simulink model "untitled"  (R2018a)
settings: Solver=FixedStepDiscrete  StartTime=0.0  StopTime=100  RelTol=1e-3
values from neighbouring files (symbols this model uses):
  coeff = randi([0, 1], 3, 60)*2-1    [Untitled.m]
libraries: filter_library x261, simulink x2, dspsrcs4 x1
(part 1 of 2)
settings Model: Creator=Orion  LastModifiedBy=Orion
settings OptimizationCC: BlockReduction=off  ConditionallyExecuteInputs=off  DefaultParameterBehavior=Inlined
settings DebuggingCC: AlgebraicLoopMsg=error  SingleTaskRateTransMsg=error
settings HardwareCC: ProdBitPerPointer=32  ProdBitPerSizeT=32  ProdBitPerPtrDiffT=32  ProdLargestAtomicFloat=None  ProdIntDivRoundTo=Undefined  ProdEndianess=Unspecified  ProdWordSize=32  ProdHWDeviceType=ASIC/FPGA->ASIC/FPGA  TargetBitPerPointer=64  TargetBitPerSizeT=64  TargetBitPerPtrDiffT=64  TargetLongLongMode=on  TargetIntDivRoundTo=Zero  TargetEndianess=LittleEndian  TargetWordSize=64  TargetHWDeviceType=Custom Processor->MATLAB Host Computer  ProdEqTarget=off

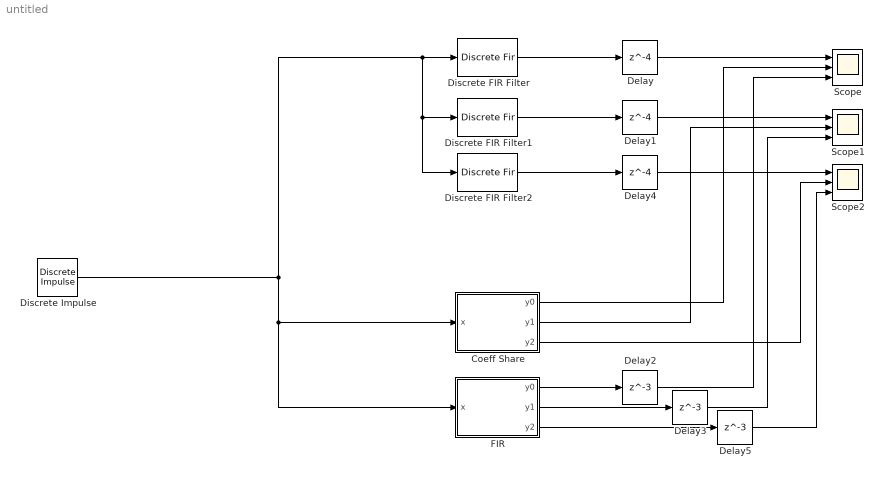
== system untitled ==
  Coeff Share : Subsystem
  Delay : Delay  DelayLength=4  InitialCondition=0
  Delay1 : Delay  DelayLength=4  InitialCondition=0
  Delay2 : Delay  DelayLength=3  InitialCondition=0
  Delay3 : Delay  DelayLength=3  InitialCondition=0
  Delay4 : Delay  DelayLength=4  InitialCondition=0
  Delay5 : Delay  DelayLength=3  InitialCondition=0
  Discrete Impulse : dspsrcs4/Discrete  Impulse  Delay=0  SampleTime=1  FrameSample=1  OutputFrames=off  dataType=Fixed-point  isSigned=on  wordLen=12  udDataType=sfix(16)  fracBitsMode=User-defined  numFracBits=11  OutDataTypeStr=fixdt(1,12,11)  LastOutDataTypeStr=fixdt(1,12,11)
  Discrete FIR Filter : DiscreteFir  Coefficients=coeff(1, :)
  Discrete FIR Filter1 : DiscreteFir  Coefficients=coeff(2, :)
  Discrete FIR Filter2 : DiscreteFir  Coefficients=coeff(3, :)
  FIR : Subsystem
  Scope : Scope  NumInputPorts=3
  Scope1 : Scope  NumInputPorts=3
  Scope2 : Scope  NumInputPorts=3
  wires:
  Discrete Impulse/1 -> FIR/1(x), Coeff Share/1(x), Discrete FIR Filter2/1, Discrete FIR Filter1/1, Discrete FIR Filter/1
  Discrete FIR Filter/1 -> Delay/1
  Delay/1 -> Scope/1
  Discrete FIR Filter1/1 -> Delay1/1
  Delay1/1 -> Scope1/1
  Coeff Share/1(y0) -> Scope/2
  Coeff Share/2(y1) -> Scope1/2
  FIR/1(y0) -> Delay2/1
  FIR/2(y1) -> Delay3/1
  Delay2/1 -> Scope/3
  Delay3/1 -> Scope1/3
  Discrete FIR Filter2/1 -> Delay4/1
  Delay4/1 -> Scope2/1
  Coeff Share/3(y2) -> Scope2/2
  FIR/3(y2) -> Delay5/1
  Delay5/1 -> Scope2/3

== system untitled/Coeff Share ==
  x : Inport
  Filter 0 : Subsystem
  Filter 1 : Subsystem
  Filter 2 : Subsystem
  Multiply-Accumulate 0 : Subsystem
  Multiply-Accumulate 1 : Subsystem
  Multiply-Accumulate 2 : Subsystem
  Multiply-Accumulate 3 : Subsystem
  Multiply-Accumulate 4 : Subsystem
  Multiply-Accumulate 5 : Subsystem
  Multiply-Accumulate 6 : Subsystem
  Multiply-Accumulate 7 : Subsystem
  Mux : Mux  Inputs=8
  Tapped Delay Line : simulink/Discrete/Tapped Delay  vinit=0.0  samptime=-1  NumDelays=60  DelayOrder=Newest  includeCurrent=off
  y0 : Outport
  y1 : Outport  Port=2
  y2 : Outport  Port=3
  wires:
  x/1 -> Tapped Delay Line/1
  Tapped Delay Line/1 -> Multiply-Accumulate 0/1(x), Multiply-Accumulate 1/1(x), Multiply-Accumulate 2/1(x), Multiply-Accumulate 3/1(x), Multiply-Accumulate 4/1(x), Multiply-Accumulate 5/1(x), Multiply-Accumulate 6/1(x), Multiply-Accumulate 7/1(x)
  Multiply-Accumulate 0/1(y) -> Mux/1
  Multiply-Accumulate 1/1(y) -> Mux/2
  Multiply-Accumulate 2/1(y) -> Mux/3
  Multiply-Accumulate 3/1(y) -> Mux/4
  Multiply-Accumulate 4/1(y) -> Mux/5
  Multiply-Accumulate 5/1(y) -> Mux/6
  Multiply-Accumulate 6/1(y) -> Mux/7
  Multiply-Accumulate 7/1(y) -> Mux/8
  Mux/1 -> Filter 0/1(data_in), Filter 1/1(data_in), Filter 2/1(data_in)
  Filter 0/1(data_out) -> y0/1
  Filter 1/1(data_out) -> y1/1
  Filter 2/1(data_out) -> y2/1

== system untitled/FIR ==
  x : Inport
  Multiply-Accumulate 1 : Subsystem
  Multiply-Accumulate 2 : Subsystem
  Multiply-Accumulate 3 : Subsystem
  Tapped Delay Line : simulink/Discrete/Tapped Delay  vinit=0.0  samptime=-1  NumDelays=60  DelayOrder=Newest  includeCurrent=off
  y0 : Outport
  y1 : Outport  Port=2
  y2 : Outport  Port=3
  wires:
  x/1 -> Tapped Delay Line/1
  Tapped Delay Line/1 -> Multiply-Accumulate 1/1(x), Multiply-Accumulate 2/1(x), Multiply-Accumulate 3/1(x)
  Multiply-Accumulate 1/1(y) -> y0/1
  Multiply-Accumulate 2/1(y) -> y1/1
  Multiply-Accumulate 3/1(y) -> y2/1

== system untitled/Coeff Share/Filter 0 ==
  data_in : Inport
  Demux : Demux  Outputs=8
  add_delay1_{1..4} (4 alike) : filter_library/Add and Delay  Inputs=++
      settings: SourceProductName=Filter Library
  add_delay2_1 : filter_library/Add and Delay  Inputs=++
      settings: SourceProductName=Filter Library
  add_delay2_2 : filter_library/Add and Delay  Inputs=++
      settings: SourceProductName=Filter Library
  add_delay3_1 : filter_library/Add and Delay  Inputs=++
      settings: SourceProductName=Filter Library
  data_out : Outport
  wires:
  add_delay1_1/1 -> add_delay2_1/1
  add_delay1_2/1 -> add_delay2_1/2
  add_delay1_3/1 -> add_delay2_2/1
  add_delay1_4/1 -> add_delay2_2/2
  add_delay2_1/1 -> add_delay3_1/1
  add_delay2_2/1 -> add_delay3_1/2
  Demux/1 -> add_delay1_1/1
  Demux/2 -> add_delay1_1/2
  Demux/3 -> add_delay1_2/1
  Demux/4 -> add_delay1_2/2
  Demux/5 -> add_delay1_3/1
  Demux/6 -> add_delay1_3/2
  Demux/7 -> add_delay1_4/1
  Demux/8 -> add_delay1_4/2
  add_delay3_1/1 -> data_out/1
  data_in/1 -> Demux/1

== system untitled/Coeff Share/Filter 1 ==
  data_in : Inport
  Demux : Demux  Outputs=8
  add_delay1_1 : filter_library/Add and Delay  Inputs=++
      settings: SourceProductName=Filter Library
  add_delay1_2 : filter_library/Add and Delay  Inputs=--
      settings: SourceProductName=Filter Library
  add_delay1_3 : filter_library/Add and Delay  Inputs=--
      settings: SourceProductName=Filter Library
  add_delay1_4 : filter_library/Add and Delay  Inputs=++
      settings: SourceProductName=Filter Library
  add_delay2_1 : filter_library/Add and Delay  Inputs=++
      settings: SourceProductName=Filter Library
  add_delay2_2 : filter_library/Add and Delay  Inputs=++
      settings: SourceProductName=Filter Library
  add_delay3_1 : filter_library/Add and Delay  Inputs=++
      settings: SourceProductName=Filter Library
  data_out : Outport
  wires:
  add_delay1_1/1 -> add_delay2_1/1
  add_delay1_2/1 -> add_delay2_1/2
  add_delay1_3/1 -> add_delay2_2/1
  add_delay1_4/1 -> add_delay2_2/2
  add_delay2_1/1 -> add_delay3_1/1
  add_delay2_2/1 -> add_delay3_1/2
  Demux/1 -> add_delay1_1/1
  Demux/2 -> add_delay1_1/2
  Demux/3 -> add_delay1_2/1
  Demux/4 -> add_delay1_2/2
  Demux/5 -> add_delay1_3/1
  Demux/6 -> add_delay1_3/2
  Demux/7 -> add_delay1_4/1
  Demux/8 -> add_delay1_4/2
  add_delay3_1/1 -> data_out/1
  data_in/1 -> Demux/1

== system untitled/Coeff Share/Filter 2 ==
  data_in : Inport
  Demux : Demux  Outputs=8
  add_delay1_1 : filter_library/Add and Delay  Inputs=+-
      settings: SourceProductName=Filter Library
  add_delay1_2 : filter_library/Add and Delay  Inputs=+-
      settings: SourceProductName=Filter Library
  add_delay1_3 : filter_library/Add and Delay  Inputs=-+
      settings: SourceProductName=Filter Library
  add_delay1_4 : filter_library/Add and Delay  Inputs=-+
      settings: SourceProductName=Filter Library
  add_delay2_1 : filter_library/Add and Delay  Inputs=++
      settings: SourceProductName=Filter Library
  add_delay2_2 : filter_library/Add and Delay  Inputs=++
      settings: SourceProductName=Filter Library
  add_delay3_1 : filter_library/Add and Delay  Inputs=++
      settings: SourceProductName=Filter Library
  data_out : Outport
  wires:
  add_delay1_1/1 -> add_delay2_1/1
  add_delay1_2/1 -> add_delay2_1/2
  add_delay1_3/1 -> add_delay2_2/1
  add_delay1_4/1 -> add_delay2_2/2
  add_delay2_1/1 -> add_delay3_1/1
  add_delay2_2/1 -> add_delay3_1/2
  Demux/1 -> add_delay1_1/1
  Demux/2 -> add_delay1_1/2
  Demux/3 -> add_delay1_2/1
  Demux/4 -> add_delay1_2/2
  Demux/5 -> add_delay1_3/1
  Demux/6 -> add_delay1_3/2
  Demux/7 -> add_delay1_4/1
  Demux/8 -> add_delay1_4/2
  add_delay3_1/1 -> data_out/1
  data_in/1 -> Demux/1

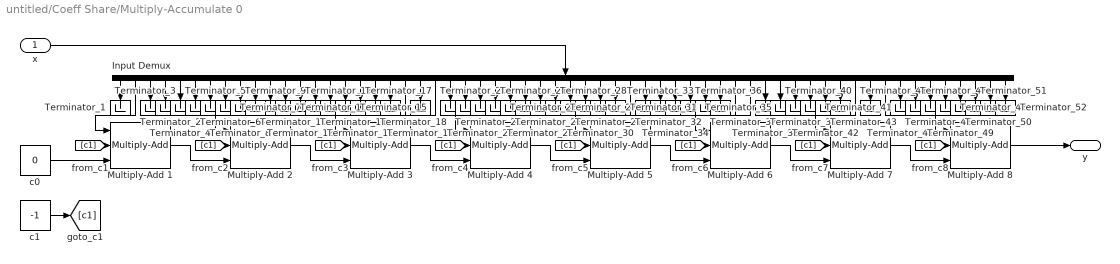
== system untitled/Coeff Share/Multiply-Accumulate 0 ==
  x : Inport
  Input Demux : Demux  Outputs=60
  Multiply-Add {1..8} (8 alike) : filter_library/Multiply-Add  SystemSampleTime=-1
      settings: SourceProductName=Filter Library
  Terminator_{1..52} (52 alike) : Terminator
  c0 : Constant  Value=0  OutDataTypeStr=fixdt(1, 12, 7)  SampleTime=1
  c1 : Constant  Value=-1  OutDataTypeStr=fixdt(1, 12, 7)  SampleTime=1
  y : Outport
  wires:
  [c1] -> Multiply-Add 1/2
  [c1] -> Multiply-Add 2/2
  [c1] -> Multiply-Add 3/2
  [c1] -> Multiply-Add 4/2
  [c1] -> Multiply-Add 5/2
  [c1] -> Multiply-Add 6/2
  [c1] -> Multiply-Add 7/2
  [c1] -> Multiply-Add 8/2
  Multiply-Add 1/1 -> Multiply-Add 2/3
  Multiply-Add 2/1 -> Multiply-Add 3/3
  Multiply-Add 3/1 -> Multiply-Add 4/3
  Multiply-Add 4/1 -> Multiply-Add 5/3
  Multiply-Add 5/1 -> Multiply-Add 6/3
  Multiply-Add 6/1 -> Multiply-Add 7/3
  Multiply-Add 7/1 -> Multiply-Add 8/3
  Multiply-Add 8/1 -> y/1
  x/1 -> Input Demux/1
  Input Demux/2 -> Multiply-Add 1/1
  Input Demux/20 -> Multiply-Add 2/1
  Input Demux/22 -> Multiply-Add 3/1
  Input Demux/35 -> Multiply-Add 4/1
  Input Demux/42 -> Multiply-Add 5/1
  Input Demux/43 -> Multiply-Add 6/1
  Input Demux/50 -> Multiply-Add 7/1
  Input Demux/52 -> Multiply-Add 8/1
  c1/1 -> [c1]
  c0/1 -> Multiply-Add 1/3
  Input Demux/1 -> Terminator_1/1
  Input Demux/3 -> Terminator_2/1
  Input Demux/4 -> Terminator_3/1
  Input Demux/5 -> Terminator_4/1
  Input Demux/6 -> Terminator_5/1
  Input Demux/7 -> Terminator_6/1
  Input Demux/8 -> Terminator_7/1
  Input Demux/9 -> Terminator_8/1
  Input Demux/10 -> Terminator_9/1
  Input Demux/11 -> Terminator_10/1
  Input Demux/12 -> Terminator_11/1
  Input Demux/13 -> Terminator_12/1
  Input Demux/14 -> Terminator_13/1
  Input Demux/15 -> Terminator_14/1
  Input Demux/16 -> Terminator_15/1
  Input Demux/17 -> Terminator_16/1
  Input Demux/18 -> Terminator_17/1
  Input Demux/19 -> Terminator_18/1
  Input Demux/21 -> Terminator_19/1
  Input Demux/23 -> Terminator_20/1
  Input Demux/24 -> Terminator_21/1
  Input Demux/25 -> Terminator_22/1
  Input Demux/26 -> Terminator_23/1
  Input Demux/27 -> Terminator_24/1
  Input Demux/28 -> Terminator_25/1
  Input Demux/29 -> Terminator_26/1
  Input Demux/30 -> Terminator_27/1
  Input Demux/31 -> Terminator_28/1
  Input Demux/32 -> Terminator_29/1
  Input Demux/33 -> Terminator_30/1
  Input Demux/34 -> Terminator_31/1
  Input Demux/36 -> Terminator_32/1
  Input Demux/37 -> Terminator_33/1
  Input Demux/38 -> Terminator_34/1
  Input Demux/39 -> Terminator_35/1
  Input Demux/40 -> Terminator_36/1
  Input Demux/41 -> Terminator_37/1
  Input Demux/44 -> Terminator_38/1
  Input Demux/45 -> Terminator_39/1
  Input Demux/46 -> Terminator_40/1
  Input Demux/47 -> Terminator_41/1
  Input Demux/48 -> Terminator_42/1
  Input Demux/49 -> Terminator_43/1
  Input Demux/51 -> Terminator_44/1
  Input Demux/53 -> Terminator_45/1
  Input Demux/54 -> Terminator_46/1
  Input Demux/55 -> Terminator_47/1
  Input Demux/56 -> Terminator_48/1
  Input Demux/57 -> Terminator_49/1
  Input Demux/58 -> Terminator_50/1
  Input Demux/59 -> Terminator_51/1
  Input Demux/60 -> Terminator_52/1

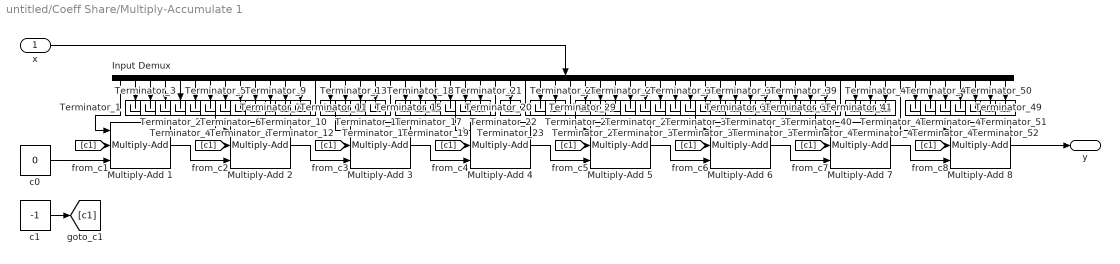
== system untitled/Coeff Share/Multiply-Accumulate 1 ==
  x : Inport
  Input Demux : Demux  Outputs=60
  Multiply-Add {1..8} (8 alike) : filter_library/Multiply-Add  SystemSampleTime=-1
      settings: SourceProductName=Filter Library
  Terminator_{1..52} (52 alike) : Terminator
  c0 : Constant  Value=0  OutDataTypeStr=fixdt(1, 12, 7)  SampleTime=1
  c1 : Constant  Value=-1  OutDataTypeStr=fixdt(1, 12, 7)  SampleTime=1
  y : Outport
  wires:
  [c1] -> Multiply-Add 1/2
  [c1] -> Multiply-Add 2/2
  [c1] -> Multiply-Add 3/2
  [c1] -> Multiply-Add 4/2
  [c1] -> Multiply-Add 5/2
  [c1] -> Multiply-Add 6/2
  [c1] -> Multiply-Add 7/2
  [c1] -> Multiply-Add 8/2
  Multiply-Add 1/1 -> Multiply-Add 2/3
  Multiply-Add 2/1 -> Multiply-Add 3/3
  Multiply-Add 3/1 -> Multiply-Add 4/3
  Multiply-Add 4/1 -> Multiply-Add 5/3
  Multiply-Add 5/1 -> Multiply-Add 6/3
  Multiply-Add 6/1 -> Multiply-Add 7/3
  Multiply-Add 7/1 -> Multiply-Add 8/3
  Multiply-Add 8/1 -> y/1
  x/1 -> Input Demux/1
  Input Demux/1 -> Multiply-Add 1/1
  Input Demux/14 -> Multiply-Add 2/1
  Input Demux/19 -> Multiply-Add 3/1
  Input Demux/26 -> Multiply-Add 4/1
  Input Demux/28 -> Multiply-Add 5/1
  Input Demux/31 -> Multiply-Add 6/1
  Input Demux/49 -> Multiply-Add 7/1
  Input Demux/53 -> Multiply-Add 8/1
  c1/1 -> [c1]
  c0/1 -> Multiply-Add 1/3
  Input Demux/2 -> Terminator_1/1
  Input Demux/3 -> Terminator_2/1
  Input Demux/4 -> Terminator_3/1
  Input Demux/5 -> Terminator_4/1
  Input Demux/6 -> Terminator_5/1
  Input Demux/7 -> Terminator_6/1
  Input Demux/8 -> Terminator_7/1
  Input Demux/9 -> Terminator_8/1
  Input Demux/10 -> Terminator_9/1
  Input Demux/11 -> Terminator_10/1
  Input Demux/12 -> Terminator_11/1
  Input Demux/13 -> Terminator_12/1
  Input Demux/15 -> Terminator_13/1
  Input Demux/16 -> Terminator_14/1
  Input Demux/17 -> Terminator_15/1
  Input Demux/18 -> Terminator_16/1
  Input Demux/20 -> Terminator_17/1
  Input Demux/21 -> Terminator_18/1
  Input Demux/22 -> Terminator_19/1
  Input Demux/23 -> Terminator_20/1
  Input Demux/24 -> Terminator_21/1
  Input Demux/25 -> Terminator_22/1
  Input Demux/27 -> Terminator_23/1
  Input Demux/29 -> Terminator_24/1
  Input Demux/30 -> Terminator_25/1
  Input Demux/32 -> Terminator_26/1
  Input Demux/33 -> Terminator_27/1
  Input Demux/34 -> Terminator_28/1
  Input Demux/35 -> Terminator_29/1
  Input Demux/36 -> Terminator_30/1
  Input Demux/37 -> Terminator_31/1
  Input Demux/38 -> Terminator_32/1
  Input Demux/39 -> Terminator_33/1
  Input Demux/40 -> Terminator_34/1
  Input Demux/41 -> Terminator_35/1
  Input Demux/42 -> Terminator_36/1
  Input Demux/43 -> Terminator_37/1
  Input Demux/44 -> Terminator_38/1
  Input Demux/45 -> Terminator_39/1
  Input Demux/46 -> Terminator_40/1
  Input Demux/47 -> Terminator_41/1
  Input Demux/48 -> Terminator_42/1
  Input Demux/50 -> Terminator_43/1
  Input Demux/51 -> Terminator_44/1
  Input Demux/52 -> Terminator_45/1
  Input Demux/54 -> Terminator_46/1
  Input Demux/55 -> Terminator_47/1
  Input Demux/56 -> Terminator_48/1
  Input Demux/57 -> Terminator_49/1
  Input Demux/58 -> Terminator_50/1
  Input Demux/59 -> Terminator_51/1
  Input Demux/60 -> Terminator_52/1

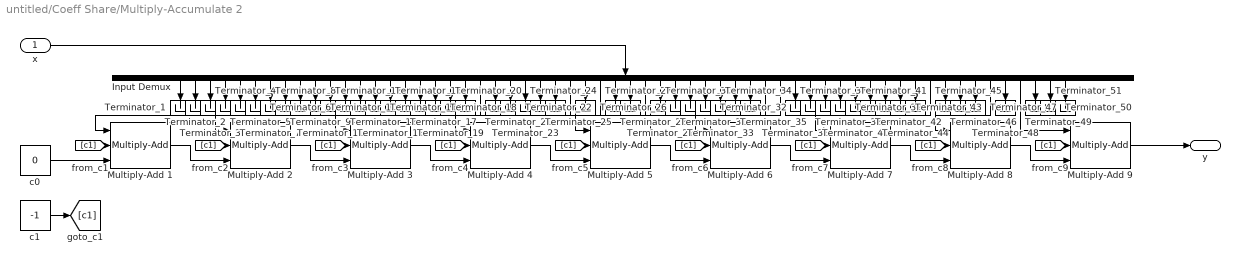
== system untitled/Coeff Share/Multiply-Accumulate 2 ==
  x : Inport
  Input Demux : Demux  Outputs=60
  Multiply-Add {1..9} (9 alike) : filter_library/Multiply-Add  SystemSampleTime=-1
      settings: SourceProductName=Filter Library
  Terminator_{1..51} (51 alike) : Terminator
  c0 : Constant  Value=0  OutDataTypeStr=fixdt(1, 12, 7)  SampleTime=1
  c1 : Constant  Value=-1  OutDataTypeStr=fixdt(1, 12, 7)  SampleTime=1
  y : Outport
  wires:
  [c1] -> Multiply-Add 1/2
  [c1] -> Multiply-Add 2/2
  [c1] -> Multiply-Add 3/2
  [c1] -> Multiply-Add 4/2
  [c1] -> Multiply-Add 5/2
  [c1] -> Multiply-Add 6/2
  [c1] -> Multiply-Add 7/2
  [c1] -> Multiply-Add 8/2
  [c1] -> Multiply-Add 9/2
  Multiply-Add 1/1 -> Multiply-Add 2/3
  Multiply-Add 2/1 -> Multiply-Add 3/3
  Multiply-Add 3/1 -> Multiply-Add 4/3
  Multiply-Add 4/1 -> Multiply-Add 5/3
  Multiply-Add 5/1 -> Multiply-Add 6/3
  Multiply-Add 6/1 -> Multiply-Add 7/3
  Multiply-Add 7/1 -> Multiply-Add 8/3
  Multiply-Add 8/1 -> Multiply-Add 9/3
  Multiply-Add 9/1 -> y/1
  x/1 -> Input Demux/1
  Input Demux/21 -> Multiply-Add 1/1
  Input Demux/27 -> Multiply-Add 2/1
  Input Demux/29 -> Multiply-Add 3/1
  Input Demux/32 -> Multiply-Add 4/1
  Input Demux/40 -> Multiply-Add 5/1
  Input Demux/41 -> Multiply-Add 6/1
  Input Demux/51 -> Multiply-Add 7/1
  Input Demux/55 -> Multiply-Add 8/1
  Input Demux/57 -> Multiply-Add 9/1
  c1/1 -> [c1]
  c0/1 -> Multiply-Add 1/3
  Input Demux/1 -> Terminator_1/1
  Input Demux/2 -> Terminator_2/1
  Input Demux/3 -> Terminator_3/1
  Input Demux/4 -> Terminator_4/1
  Input Demux/5 -> Terminator_5/1
  Input Demux/6 -> Terminator_6/1
  Input Demux/7 -> Terminator_7/1
  Input Demux/8 -> Terminator_8/1
  Input Demux/9 -> Terminator_9/1
  Input Demux/10 -> Terminator_10/1
  Input Demux/11 -> Terminator_11/1
  Input Demux/12 -> Terminator_12/1
  Input Demux/13 -> Terminator_13/1
  Input Demux/14 -> Terminator_14/1
  Input Demux/15 -> Terminator_15/1
  Input Demux/16 -> Terminator_16/1
  Input Demux/17 -> Terminator_17/1
  Input Demux/18 -> Terminator_18/1
  Input Demux/19 -> Terminator_19/1
  Input Demux/20 -> Terminator_20/1
  Input Demux/22 -> Terminator_21/1
  Input Demux/23 -> Terminator_22/1
  Input Demux/24 -> Terminator_23/1
  Input Demux/25 -> Terminator_24/1
  Input Demux/26 -> Terminator_25/1
  Input Demux/28 -> Terminator_26/1
  Input Demux/30 -> Terminator_27/1
  Input Demux/31 -> Terminator_28/1
  Input Demux/33 -> Terminator_29/1
  Input Demux/34 -> Terminator_30/1
  Input Demux/35 -> Terminator_31/1
  Input Demux/36 -> Terminator_32/1
  Input Demux/37 -> Terminator_33/1
  Input Demux/38 -> Terminator_34/1
  Input Demux/39 -> Terminator_35/1
  Input Demux/42 -> Terminator_36/1
  Input Demux/43 -> Terminator_37/1
  Input Demux/44 -> Terminator_38/1
  Input Demux/45 -> Terminator_39/1
  Input Demux/46 -> Terminator_40/1
  Input Demux/47 -> Terminator_41/1
  Input Demux/48 -> Terminator_42/1
  Input Demux/49 -> Terminator_43/1
  Input Demux/50 -> Terminator_44/1
  Input Demux/52 -> Terminator_45/1
  Input Demux/53 -> Terminator_46/1
  Input Demux/54 -> Terminator_47/1
  Input Demux/56 -> Terminator_48/1
  Input Demux/58 -> Terminator_49/1
  Input Demux/59 -> Terminator_50/1
  Input Demux/60 -> Terminator_51/1

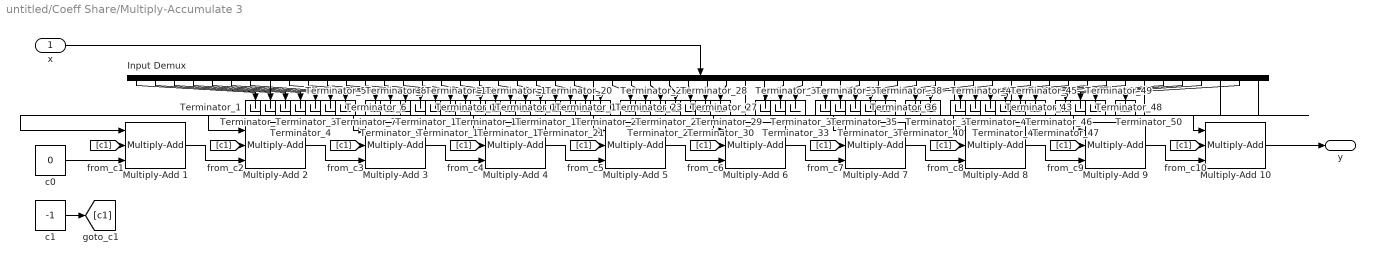
== system untitled/Coeff Share/Multiply-Accumulate 3 ==
  x : Inport
  Input Demux : Demux  Outputs=60
  Multiply-Add {1..10} (10 alike) : filter_library/Multiply-Add  SystemSampleTime=-1
      settings: SourceProductName=Filter Library
  Terminator_{1..50} (50 alike) : Terminator
  c0 : Constant  Value=0  OutDataTypeStr=fixdt(1, 12, 7)  SampleTime=1
  c1 : Constant  Value=-1  OutDataTypeStr=fixdt(1, 12, 7)  SampleTime=1
  y : Outport
  wires:
  [c1] -> Multiply-Add 1/2
  [c1] -> Multiply-Add 2/2
  [c1] -> Multiply-Add 3/2
  [c1] -> Multiply-Add 4/2
  [c1] -> Multiply-Add 5/2
  [c1] -> Multiply-Add 6/2
  [c1] -> Multiply-Add 7/2
  [c1] -> Multiply-Add 8/2
  [c1] -> Multiply-Add 9/2
  [c1] -> Multiply-Add 10/2
  Multiply-Add 1/1 -> Multiply-Add 2/3
  Multiply-Add 2/1 -> Multiply-Add 3/3
  Multiply-Add 3/1 -> Multiply-Add 4/3
  Multiply-Add 4/1 -> Multiply-Add 5/3
  Multiply-Add 5/1 -> Multiply-Add 6/3
  Multiply-Add 6/1 -> Multiply-Add 7/3
  Multiply-Add 7/1 -> Multiply-Add 8/3
  Multiply-Add 8/1 -> Multiply-Add 9/3
  Multiply-Add 9/1 -> Multiply-Add 10/3
  Multiply-Add 10/1 -> y/1
  x/1 -> Input Demux/1
  Input Demux/8 -> Multiply-Add 1/1
  Input Demux/25 -> Multiply-Add 2/1
  Input Demux/33 -> Multiply-Add 3/1
  Input Demux/34 -> Multiply-Add 4/1
  Input Demux/38 -> Multiply-Add 5/1
  Input Demux/44 -> Multiply-Add 6/1
  Input Demux/47 -> Multiply-Add 7/1
  Input Demux/54 -> Multiply-Add 8/1
  Input Demux/58 -> Multiply-Add 9/1
  Input Demux/60 -> Multiply-Add 10/1
  c1/1 -> [c1]
  c0/1 -> Multiply-Add 1/3
  Input Demux/1 -> Terminator_1/1
  Input Demux/2 -> Terminator_2/1
  Input Demux/3 -> Terminator_3/1
  Input Demux/4 -> Terminator_4/1
  Input Demux/5 -> Terminator_5/1
  Input Demux/6 -> Terminator_6/1
  Input Demux/7 -> Terminator_7/1
  Input Demux/9 -> Terminator_8/1
  Input Demux/10 -> Terminator_9/1
  Input Demux/11 -> Terminator_10/1
  Input Demux/12 -> Terminator_11/1
  Input Demux/13 -> Terminator_12/1
  Input Demux/14 -> Terminator_13/1
  Input Demux/15 -> Terminator_14/1
  Input Demux/16 -> Terminator_15/1
  Input Demux/17 -> Terminator_16/1
  Input Demux/18 -> Terminator_17/1
  Input Demux/19 -> Terminator_18/1
  Input Demux/20 -> Terminator_19/1
  Input Demux/21 -> Terminator_20/1
  Input Demux/22 -> Terminator_21/1
  Input Demux/23 -> Terminator_22/1
  Input Demux/24 -> Terminator_23/1
  Input Demux/26 -> Terminator_24/1
  Input Demux/27 -> Terminator_25/1
  Input Demux/28 -> Terminator_26/1
  Input Demux/29 -> Terminator_27/1
  Input Demux/30 -> Terminator_28/1
  Input Demux/31 -> Terminator_29/1
  Input Demux/32 -> Terminator_30/1
  Input Demux/35 -> Terminator_31/1
  Input Demux/36 -> Terminator_32/1
  Input Demux/37 -> Terminator_33/1
  Input Demux/39 -> Terminator_34/1
  Input Demux/40 -> Terminator_35/1
  Input Demux/41 -> Terminator_36/1
  Input Demux/42 -> Terminator_37/1
  Input Demux/43 -> Terminator_38/1
  Input Demux/45 -> Terminator_39/1
  Input Demux/46 -> Terminator_40/1
  Input Demux/48 -> Terminator_41/1
  Input Demux/49 -> Terminator_42/1
  Input Demux/50 -> Terminator_43/1
  Input Demux/51 -> Terminator_44/1
  Input Demux/52 -> Terminator_45/1
  Input Demux/53 -> Terminator_46/1
  Input Demux/55 -> Terminator_47/1
  Input Demux/56 -> Terminator_48/1
  Input Demux/57 -> Terminator_49/1
  Input Demux/59 -> Terminator_50/1

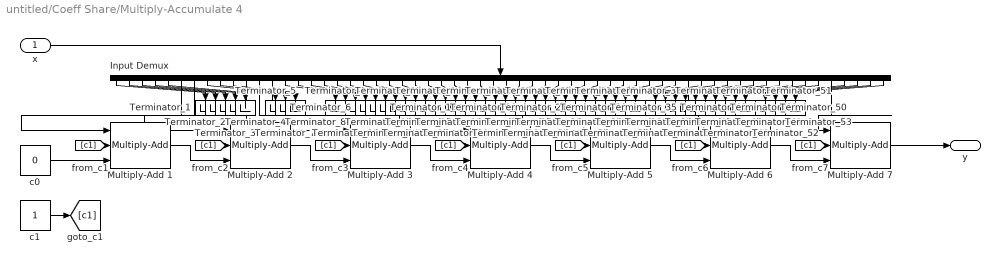
== system untitled/Coeff Share/Multiply-Accumulate 4 ==
  x : Inport
  Input Demux : Demux  Outputs=60
  Multiply-Add {1..7} (7 alike) : filter_library/Multiply-Add  SystemSampleTime=-1
      settings: SourceProductName=Filter Library
  Terminator_{1..53} (53 alike) : Terminator
  c0 : Constant  Value=0  OutDataTypeStr=fixdt(1, 12, 7)  SampleTime=1
  c1 : Constant  OutDataTypeStr=fixdt(1, 12, 7)  SampleTime=1
  y : Outport
  wires:
  [c1] -> Multiply-Add 1/2
  [c1] -> Multiply-Add 2/2
  [c1] -> Multiply-Add 3/2
  [c1] -> Multiply-Add 4/2
  [c1] -> Multiply-Add 5/2
  [c1] -> Multiply-Add 6/2
  [c1] -> Multiply-Add 7/2
  Multiply-Add 1/1 -> Multiply-Add 2/3
  Multiply-Add 2/1 -> Multiply-Add 3/3
  Multiply-Add 3/1 -> Multiply-Add 4/3
  Multiply-Add 4/1 -> Multiply-Add 5/3
  Multiply-Add 5/1 -> Multiply-Add 6/3
  Multiply-Add 6/1 -> Multiply-Add 7/3
  Multiply-Add 7/1 -> y/1
  x/1 -> Input Demux/1
  Input Demux/6 -> Multiply-Add 1/1
  Input Demux/7 -> Multiply-Add 2/1
  Input Demux/11 -> Multiply-Add 3/1
  Input Demux/12 -> Multiply-Add 4/1
  Input Demux/13 -> Multiply-Add 5/1
  Input Demux/45 -> Multiply-Add 6/1
  Input Demux/56 -> Multiply-Add 7/1
  c1/1 -> [c1]
  c0/1 -> Multiply-Add 1/3
  Input Demux/1 -> Terminator_1/1
  Input Demux/2 -> Terminator_2/1
  Input Demux/3 -> Terminator_3/1
  Input Demux/4 -> Terminator_4/1
  Input Demux/5 -> Terminator_5/1
  Input Demux/8 -> Terminator_6/1
  Input Demux/9 -> Terminator_7/1
  Input Demux/10 -> Terminator_8/1
  Input Demux/14 -> Terminator_9/1
  Input Demux/15 -> Terminator_10/1
  Input Demux/16 -> Terminator_11/1
  Input Demux/17 -> Terminator_12/1
  Input Demux/18 -> Terminator_13/1
  Input Demux/19 -> Terminator_14/1
  Input Demux/20 -> Terminator_15/1
  Input Demux/21 -> Terminator_16/1
  Input Demux/22 -> Terminator_17/1
  Input Demux/23 -> Terminator_18/1
  Input Demux/24 -> Terminator_19/1
  Input Demux/25 -> Terminator_20/1
  Input Demux/26 -> Terminator_21/1
  Input Demux/27 -> Terminator_22/1
  Input Demux/28 -> Terminator_23/1
  Input Demux/29 -> Terminator_24/1
  Input Demux/30 -> Terminator_25/1
  Input Demux/31 -> Terminator_26/1
  Input Demux/32 -> Terminator_27/1
  Input Demux/33 -> Terminator_28/1
  Input Demux/34 -> Terminator_29/1
  Input Demux/35 -> Terminator_30/1
  Input Demux/36 -> Terminator_31/1
  Input Demux/37 -> Terminator_32/1
  Input Demux/38 -> Terminator_33/1
  Input Demux/39 -> Terminator_34/1
  Input Demux/40 -> Terminator_35/1
  Input Demux/41 -> Terminator_36/1
  Input Demux/42 -> Terminator_37/1
  Input Demux/43 -> Terminator_38/1
  Input Demux/44 -> Terminator_39/1
  Input Demux/46 -> Terminator_40/1
  Input Demux/47 -> Terminator_41/1
  Input Demux/48 -> Terminator_42/1
  Input Demux/49 -> Terminator_43/1
  Input Demux/50 -> Terminator_44/1
  Input Demux/51 -> Terminator_45/1
  Input Demux/52 -> Terminator_46/1
  Input Demux/53 -> Terminator_47/1
  Input Demux/54 -> Terminator_48/1
  Input Demux/55 -> Terminator_49/1
  Input Demux/57 -> Terminator_50/1
  Input Demux/58 -> Terminator_51/1
  Input Demux/59 -> Terminator_52/1
  Input Demux/60 -> Terminator_53/1

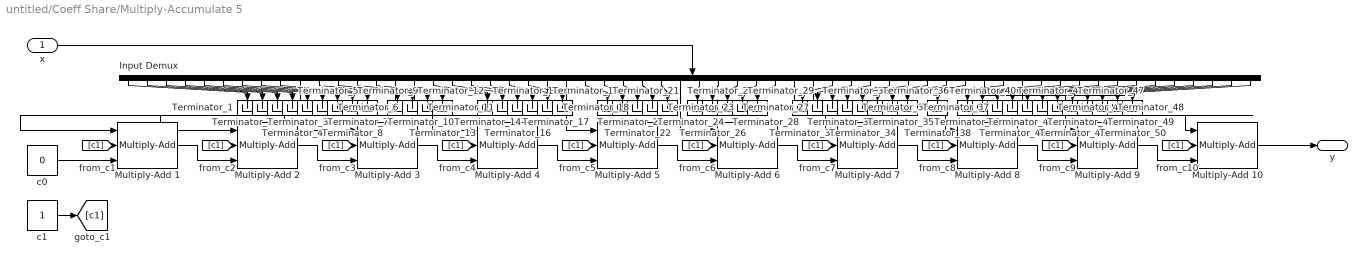
== system untitled/Coeff Share/Multiply-Accumulate 5 ==
  x : Inport
  Input Demux : Demux  Outputs=60
  Multiply-Add {1..10} (10 alike) : filter_library/Multiply-Add  SystemSampleTime=-1
      settings: SourceProductName=Filter Library
  Terminator_{1..50} (50 alike) : Terminator
  c0 : Constant  Value=0  OutDataTypeStr=fixdt(1, 12, 7)  SampleTime=1
  c1 : Constant  OutDataTypeStr=fixdt(1, 12, 7)  SampleTime=1
  y : Outport
  wires:
  [c1] -> Multiply-Add 1/2
  [c1] -> Multiply-Add 2/2
  [c1] -> Multiply-Add 3/2
  [c1] -> Multiply-Add 4/2
  [c1] -> Multiply-Add 5/2
  [c1] -> Multiply-Add 6/2
  [c1] -> Multiply-Add 7/2
  [c1] -> Multiply-Add 8/2
  [c1] -> Multiply-Add 9/2
  [c1] -> Multiply-Add 10/2
  Multiply-Add 1/1 -> Multiply-Add 2/3
  Multiply-Add 2/1 -> Multiply-Add 3/3
  Multiply-Add 3/1 -> Multiply-Add 4/3
  Multiply-Add 4/1 -> Multiply-Add 5/3
  Multiply-Add 5/1 -> Multiply-Add 6/3
  Multiply-Add 6/1 -> Multiply-Add 7/3
  Multiply-Add 7/1 -> Multiply-Add 8/3
  Multiply-Add 8/1 -> Multiply-Add 9/3
  Multiply-Add 9/1 -> Multiply-Add 10/3
  Multiply-Add 10/1 -> y/1
  x/1 -> Input Demux/1
  Input Demux/10 -> Multiply-Add 1/1
  Input Demux/15 -> Multiply-Add 2/1
  Input Demux/16 -> Multiply-Add 3/1
  Input Demux/23 -> Multiply-Add 4/1
  Input Demux/24 -> Multiply-Add 5/1
  Input Demux/30 -> Multiply-Add 6/1
  Input Demux/36 -> Multiply-Add 7/1
  Input Demux/37 -> Multiply-Add 8/1
  Input Demux/46 -> Multiply-Add 9/1
  Input Demux/48 -> Multiply-Add 10/1
  c1/1 -> [c1]
  c0/1 -> Multiply-Add 1/3
  Input Demux/1 -> Terminator_1/1
  Input Demux/2 -> Terminator_2/1
  Input Demux/3 -> Terminator_3/1
  Input Demux/4 -> Terminator_4/1
  Input Demux/5 -> Terminator_5/1
  Input Demux/6 -> Terminator_6/1
  Input Demux/7 -> Terminator_7/1
  Input Demux/8 -> Terminator_8/1
  Input Demux/9 -> Terminator_9/1
  Input Demux/11 -> Terminator_10/1
  Input Demux/12 -> Terminator_11/1
  Input Demux/13 -> Terminator_12/1
  Input Demux/14 -> Terminator_13/1
  Input Demux/17 -> Terminator_14/1
  Input Demux/18 -> Terminator_15/1
  Input Demux/19 -> Terminator_16/1
  Input Demux/20 -> Terminator_17/1
  Input Demux/21 -> Terminator_18/1
  Input Demux/22 -> Terminator_19/1
  Input Demux/25 -> Terminator_20/1
  Input Demux/26 -> Terminator_21/1
  Input Demux/27 -> Terminator_22/1
  Input Demux/28 -> Terminator_23/1
  Input Demux/29 -> Terminator_24/1
  Input Demux/31 -> Terminator_25/1
  Input Demux/32 -> Terminator_26/1
  Input Demux/33 -> Terminator_27/1
  Input Demux/34 -> Terminator_28/1
  Input Demux/35 -> Terminator_29/1
  Input Demux/38 -> Terminator_30/1
  Input Demux/39 -> Terminator_31/1
  Input Demux/40 -> Terminator_32/1
  Input Demux/41 -> Terminator_33/1
  Input Demux/42 -> Terminator_34/1
  Input Demux/43 -> Terminator_35/1
  Input Demux/44 -> Terminator_36/1
  Input Demux/45 -> Terminator_37/1
  Input Demux/47 -> Terminator_38/1
  Input Demux/49 -> Terminator_39/1
  Input Demux/50 -> Terminator_40/1
  Input Demux/51 -> Terminator_41/1
  Input Demux/52 -> Terminator_42/1
  Input Demux/53 -> Terminator_43/1
  Input Demux/54 -> Terminator_44/1
  Input Demux/55 -> Terminator_45/1
  Input Demux/56 -> Terminator_46/1
  Input Demux/57 -> Terminator_47/1
  Input Demux/58 -> Terminator_48/1
  Input Demux/59 -> Terminator_49/1
  Input Demux/60 -> Terminator_50/1

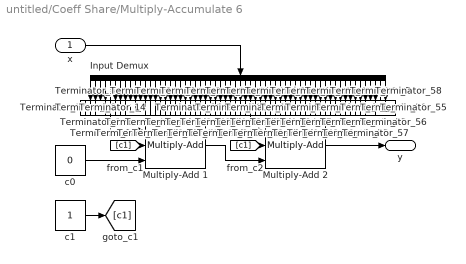
== system untitled/Coeff Share/Multiply-Accumulate 6 ==
  x : Inport
  Input Demux : Demux  Outputs=60
  Multiply-Add 1 : filter_library/Multiply-Add  SystemSampleTime=-1
      settings: SourceProductName=Filter Library
  Multiply-Add 2 : filter_library/Multiply-Add  SystemSampleTime=-1
      settings: SourceProductName=Filter Library
  Terminator_{1..58} (58 alike) : Terminator
  c0 : Constant  Value=0  OutDataTypeStr=fixdt(1, 12, 7)  SampleTime=1
  c1 : Constant  OutDataTypeStr=fixdt(1, 12, 7)  SampleTime=1
  y : Outport
  wires:
  [c1] -> Multiply-Add 1/2
  [c1] -> Multiply-Add 2/2
  Multiply-Add 1/1 -> Multiply-Add 2/3
  Multiply-Add 2/1 -> y/1
  x/1 -> Input Demux/1
  Input Demux/5 -> Multiply-Add 1/1
  Input Demux/59 -> Multiply-Add 2/1
  c1/1 -> [c1]
  c0/1 -> Multiply-Add 1/3
  Input Demux/1 -> Terminator_1/1
  Input Demux/2 -> Terminator_2/1
  Input Demux/3 -> Terminator_3/1
  Input Demux/4 -> Terminator_4/1
  Input Demux/6 -> Terminator_5/1
  Input Demux/7 -> Terminator_6/1
  Input Demux/8 -> Terminator_7/1
  Input Demux/9 -> Terminator_8/1
  Input Demux/10 -> Terminator_9/1
  Input Demux/11 -> Terminator_10/1
  Input Demux/12 -> Terminator_11/1
  Input Demux/13 -> Terminator_12/1
  Input Demux/14 -> Terminator_13/1
  Input Demux/15 -> Terminator_14/1
  Input Demux/16 -> Terminator_15/1
  Input Demux/17 -> Terminator_16/1
  Input Demux/18 -> Terminator_17/1
  Input Demux/19 -> Terminator_18/1
  Input Demux/20 -> Terminator_19/1
  Input Demux/21 -> Terminator_20/1
  Input Demux/22 -> Terminator_21/1
  Input Demux/23 -> Terminator_22/1
  Input Demux/24 -> Terminator_23/1
  Input Demux/25 -> Terminator_24/1
  Input Demux/26 -> Terminator_25/1
  Input Demux/27 -> Terminator_26/1
  Input Demux/28 -> Terminator_27/1
  Input Demux/29 -> Terminator_28/1
  Input Demux/30 -> Terminator_29/1
  Input Demux/31 -> Terminator_30/1
  Input Demux/32 -> Terminator_31/1
  Input Demux/33 -> Terminator_32/1
  Input Demux/34 -> Terminator_33/1
  Input Demux/35 -> Terminator_34/1
  Input Demux/36 -> Terminator_35/1
  Input Demux/37 -> Terminator_36/1
  Input Demux/38 -> Terminator_37/1
  Input Demux/39 -> Terminator_38/1
  Input Demux/40 -> Terminator_39/1
  Input Demux/41 -> Terminator_40/1
  Input Demux/42 -> Terminator_41/1
  Input Demux/43 -> Terminator_42/1
  Input Demux/44 -> Terminator_43/1
  Input Demux/45 -> Terminator_44/1
  Input Demux/46 -> Terminator_45/1
  Input Demux/47 -> Terminator_46/1
  Input Demux/48 -> Terminator_47/1
  Input Demux/49 -> Terminator_48/1
  Input Demux/50 -> Terminator_49/1
  Input Demux/51 -> Terminator_50/1
  Input Demux/52 -> Terminator_51/1
  Input Demux/53 -> Terminator_52/1
  Input Demux/54 -> Terminator_53/1
  Input Demux/55 -> Terminator_54/1
  Input Demux/56 -> Terminator_55/1
  Input Demux/57 -> Terminator_56/1
  Input Demux/58 -> Terminator_57/1
  Input Demux/60 -> Terminator_58/1

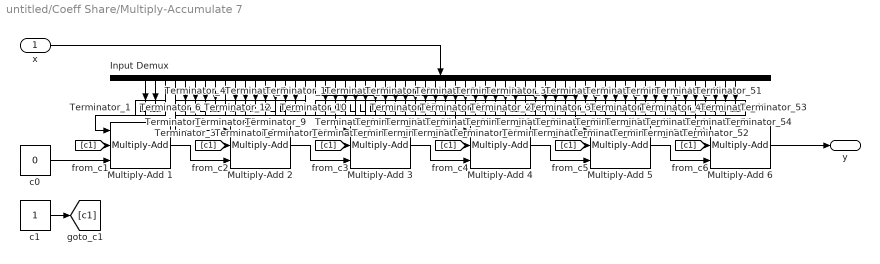
== system untitled/Coeff Share/Multiply-Accumulate 7 ==
  x : Inport
  Input Demux : Demux  Outputs=60
  Multiply-Add {1..6} (6 alike) : filter_library/Multiply-Add  SystemSampleTime=-1
      settings: SourceProductName=Filter Library
  Terminator_{1..54} (54 alike) : Terminator
  c0 : Constant  Value=0  OutDataTypeStr=fixdt(1, 12, 7)  SampleTime=1
  c1 : Constant  OutDataTypeStr=fixdt(1, 12, 7)  SampleTime=1
  y : Outport
  wires:
  [c1] -> Multiply-Add 1/2
  [c1] -> Multiply-Add 2/2
  [c1] -> Multiply-Add 3/2
  [c1] -> Multiply-Add 4/2
  [c1] -> Multiply-Add 5/2
  [c1] -> Multiply-Add 6/2
  Multiply-Add 1/1 -> Multiply-Add 2/3
  Multiply-Add 2/1 -> Multiply-Add 3/3
  Multiply-Add 3/1 -> Multiply-Add 4/3
  Multiply-Add 4/1 -> Multiply-Add 5/3
  Multiply-Add 5/1 -> Multiply-Add 6/3
  Multiply-Add 6/1 -> y/1
  x/1 -> Input Demux/1
  Input Demux/3 -> Multiply-Add 1/1
  Input Demux/4 -> Multiply-Add 2/1
  Input Demux/9 -> Multiply-Add 3/1
  Input Demux/17 -> Multiply-Add 4/1
  Input Demux/18 -> Multiply-Add 5/1
  Input Demux/39 -> Multiply-Add 6/1
  c1/1 -> [c1]
  c0/1 -> Multiply-Add 1/3
  Input Demux/1 -> Terminator_1/1
  Input Demux/2 -> Terminator_2/1
  Input Demux/5 -> Terminator_3/1
  Input Demux/6 -> Terminator_4/1
  Input Demux/7 -> Terminator_5/1
  Input Demux/8 -> Terminator_6/1
  Input Demux/10 -> Terminator_7/1
  Input Demux/11 -> Terminator_8/1
  Input Demux/12 -> Terminator_9/1
  Input Demux/13 -> Terminator_10/1
  Input Demux/14 -> Terminator_11/1
  Input Demux/15 -> Terminator_12/1
  Input Demux/16 -> Terminator_13/1
  Input Demux/19 -> Terminator_14/1
  Input Demux/20 -> Terminator_15/1
  Input Demux/21 -> Terminator_16/1
  Input Demux/22 -> Terminator_17/1
  Input Demux/23 -> Terminator_18/1
  Input Demux/24 -> Terminator_19/1
  Input Demux/25 -> Terminator_20/1
  Input Demux/26 -> Terminator_21/1
  Input Demux/27 -> Terminator_22/1
  Input Demux/28 -> Terminator_23/1
  Input Demux/29 -> Terminator_24/1
  Input Demux/30 -> Terminator_25/1
  Input Demux/31 -> Terminator_26/1
  Input Demux/32 -> Terminator_27/1
  Input Demux/33 -> Terminator_28/1
  Input Demux/34 -> Terminator_29/1
  Input Demux/35 -> Terminator_30/1
  Input Demux/36 -> Terminator_31/1
  Input Demux/37 -> Terminator_32/1
  Input Demux/38 -> Terminator_33/1
  Input Demux/40 -> Terminator_34/1
  Input Demux/41 -> Terminator_35/1
  Input Demux/42 -> Terminator_36/1
  Input Demux/43 -> Terminator_37/1
  Input Demux/44 -> Terminator_38/1
  Input Demux/45 -> Terminator_39/1
  Input Demux/46 -> Terminator_40/1
  Input Demux/47 -> Terminator_41/1
  Input Demux/48 -> Terminator_42/1
  Input Demux/49 -> Terminator_43/1
  Input Demux/50 -> Terminator_44/1
  Input Demux/51 -> Terminator_45/1
  Input Demux/52 -> Terminator_46/1
  Input Demux/53 -> Terminator_47/1
  Input Demux/54 -> Terminator_48/1
  Input Demux/55 -> Terminator_49/1
  Input Demux/56 -> Terminator_50/1
  Input Demux/57 -> Terminator_51/1
  Input Demux/58 -> Terminator_52/1
  Input Demux/59 -> Terminator_53/1
  Input Demux/60 -> Terminator_54/1

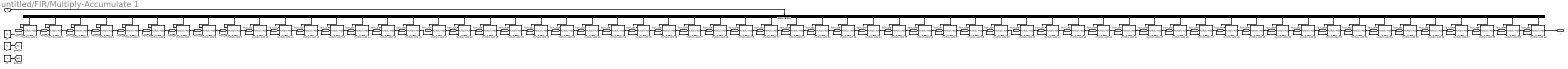
== system untitled/FIR/Multiply-Accumulate 1 ==
  x : Inport
  Input Demux : Demux  Outputs=60
  Multiply-Add {1..60} (60 alike) : filter_library/Multiply-Add  SystemSampleTime=-1
      settings: SourceProductName=Filter Library
  c0 : Constant  Value=0  OutDataTypeStr=fixdt(1, 12, 7)  SampleTime=1
  c1 : Constant  Value=-1  OutDataTypeStr=fixdt(1, 12, 7)  SampleTime=1
  c2 : Constant  OutDataTypeStr=fixdt(1, 12, 7)  SampleTime=1
  y : Outport
  wires:
  [c1] -> Multiply-Add 1/2
  [c1] -> Multiply-Add 2/2
  [c2] -> Multiply-Add 3/2
  [c2] -> Multiply-Add 4/2
  [c2] -> Multiply-Add 5/2
  [c2] -> Multiply-Add 6/2
  [c2] -> Multiply-Add 7/2
  [c1] -> Multiply-Add 8/2
  [c2] -> Multiply-Add 9/2
  [c2] -> Multiply-Add 10/2
  [c2] -> Multiply-Add 11/2
  [c2] -> Multiply-Add 12/2
  [c2] -> Multiply-Add 13/2
  [c1] -> Multiply-Add 14/2
  [c2] -> Multiply-Add 15/2
  [c2] -> Multiply-Add 16/2
  [c2] -> Multiply-Add 17/2
  [c2] -> Multiply-Add 18/2
  [c1] -> Multiply-Add 19/2
  [c1] -> Multiply-Add 20/2
  [c1] -> Multiply-Add 21/2
  [c1] -> Multiply-Add 22/2
  [c2] -> Multiply-Add 23/2
  [c2] -> Multiply-Add 24/2
  [c1] -> Multiply-Add 25/2
  [c1] -> Multiply-Add 26/2
  [c1] -> Multiply-Add 27/2
  [c1] -> Multiply-Add 28/2
  [c1] -> Multiply-Add 29/2
  [c2] -> Multiply-Add 30/2
  [c1] -> Multiply-Add 31/2
  [c1] -> Multiply-Add 32/2
  [c1] -> Multiply-Add 33/2
  [c1] -> Multiply-Add 34/2
  [c1] -> Multiply-Add 35/2
  [c2] -> Multiply-Add 36/2
  [c2] -> Multiply-Add 37/2
  [c1] -> Multiply-Add 38/2
  [c2] -> Multiply-Add 39/2
  [c1] -> Multiply-Add 40/2
  [c1] -> Multiply-Add 41/2
  [c1] -> Multiply-Add 42/2
  [c1] -> Multiply-Add 43/2
  [c1] -> Multiply-Add 44/2
  [c2] -> Multiply-Add 45/2
  [c2] -> Multiply-Add 46/2
  [c1] -> Multiply-Add 47/2
  [c2] -> Multiply-Add 48/2
  [c1] -> Multiply-Add 49/2
  [c1] -> Multiply-Add 50/2
  [c1] -> Multiply-Add 51/2
  [c1] -> Multiply-Add 52/2
  [c1] -> Multiply-Add 53/2
  [c1] -> Multiply-Add 54/2
  [c1] -> Multiply-Add 55/2
  [c2] -> Multiply-Add 56/2
  [c1] -> Multiply-Add 57/2
  [c1] -> Multiply-Add 58/2
  [c2] -> Multiply-Add 59/2
  [c1] -> Multiply-Add 60/2
  Multiply-Add 1/1 -> Multiply-Add 2/3
  Multiply-Add 2/1 -> Multiply-Add 3/3
  Multiply-Add 3/1 -> Multiply-Add 4/3
  Multiply-Add 4/1 -> Multiply-Add 5/3
  Multiply-Add 5/1 -> Multiply-Add 6/3
  Multiply-Add 6/1 -> Multiply-Add 7/3
  Multiply-Add 7/1 -> Multiply-Add 8/3
  Multiply-Add 8/1 -> Multiply-Add 9/3
  Multiply-Add 9/1 -> Multiply-Add 10/3
  Multiply-Add 10/1 -> Multiply-Add 11/3
  Multiply-Add 11/1 -> Multiply-Add 12/3
  Multiply-Add 12/1 -> Multiply-Add 13/3
  Multiply-Add 13/1 -> Multiply-Add 14/3
  Multiply-Add 14/1 -> Multiply-Add 15/3
  Multiply-Add 15/1 -> Multiply-Add 16/3
  Multiply-Add 16/1 -> Multiply-Add 17/3
  Multiply-Add 17/1 -> Multiply-Add 18/3
  Multiply-Add 18/1 -> Multiply-Add 19/3
  Multiply-Add 19/1 -> Multiply-Add 20/3
  Multiply-Add 20/1 -> Multiply-Add 21/3
  Multiply-Add 21/1 -> Multiply-Add 22/3
  Multiply-Add 22/1 -> Multiply-Add 23/3
  Multiply-Add 23/1 -> Multiply-Add 24/3
  Multiply-Add 24/1 -> Multiply-Add 25/3
  Multiply-Add 25/1 -> Multiply-Add 26/3
  Multiply-Add 26/1 -> Multiply-Add 27/3
  Multiply-Add 27/1 -> Multiply-Add 28/3
  Multiply-Add 28/1 -> Multiply-Add 29/3
  Multiply-Add 29/1 -> Multiply-Add 30/3
  Multiply-Add 30/1 -> Multiply-Add 31/3
  Multiply-Add 31/1 -> Multiply-Add 32/3
  Multiply-Add 32/1 -> Multiply-Add 33/3
  Multiply-Add 33/1 -> Multiply-Add 34/3
  Multiply-Add 34/1 -> Multiply-Add 35/3
  Multiply-Add 35/1 -> Multiply-Add 36/3
  Multiply-Add 36/1 -> Multiply-Add 37/3
  Multiply-Add 37/1 -> Multiply-Add 38/3
  Multiply-Add 38/1 -> Multiply-Add 39/3
  Multiply-Add 39/1 -> Multiply-Add 40/3
  Multiply-Add 40/1 -> Multiply-Add 41/3
  Multiply-Add 41/1 -> Multiply-Add 42/3
  Multiply-Add 42/1 -> Multiply-Add 43/3
  Multiply-Add 43/1 -> Multiply-Add 44/3
  Multiply-Add 44/1 -> Multiply-Add 45/3
  Multiply-Add 45/1 -> Multiply-Add 46/3
  Multiply-Add 46/1 -> Multiply-Add 47/3
  Multiply-Add 47/1 -> Multiply-Add 48/3
  Multiply-Add 48/1 -> Multiply-Add 49/3
  Multiply-Add 49/1 -> Multiply-Add 50/3
  Multiply-Add 50/1 -> Multiply-Add 51/3
  Multiply-Add 51/1 -> Multiply-Add 52/3
  Multiply-Add 52/1 -> Multiply-Add 53/3
  Multiply-Add 53/1 -> Multiply-Add 54/3
  Multiply-Add 54/1 -> Multiply-Add 55/3
  Multiply-Add 55/1 -> Multiply-Add 56/3
  Multiply-Add 56/1 -> Multiply-Add 57/3
  Multiply-Add 57/1 -> Multiply-Add 58/3
  Multiply-Add 58/1 -> Multiply-Add 59/3
  Multiply-Add 59/1 -> Multiply-Add 60/3
  Multiply-Add 60/1 -> y/1
  x/1 -> Input Demux/1
  Input Demux/1 -> Multiply-Add 1/1
  Input Demux/2 -> Multiply-Add 2/1
  Input Demux/3 -> Multiply-Add 3/1
  Input Demux/4 -> Multiply-Add 4/1
  Input Demux/5 -> Multiply-Add 5/1
  Input Demux/6 -> Multiply-Add 6/1
  Input Demux/7 -> Multiply-Add 7/1
  Input Demux/8 -> Multiply-Add 8/1
  Input Demux/9 -> Multiply-Add 9/1
  Input Demux/10 -> Multiply-Add 10/1
  Input Demux/11 -> Multiply-Add 11/1
  Input Demux/12 -> Multiply-Add 12/1
  Input Demux/13 -> Multiply-Add 13/1
  Input Demux/14 -> Multiply-Add 14/1
  Input Demux/15 -> Multiply-Add 15/1
  Input Demux/16 -> Multiply-Add 16/1
  Input Demux/17 -> Multiply-Add 17/1
  Input Demux/18 -> Multiply-Add 18/1
  Input Demux/19 -> Multiply-Add 19/1
  Input Demux/20 -> Multiply-Add 20/1
  Input Demux/21 -> Multiply-Add 21/1
  Input Demux/22 -> Multiply-Add 22/1
  Input Demux/23 -> Multiply-Add 23/1
  Input Demux/24 -> Multiply-Add 24/1
  Input Demux/25 -> Multiply-Add 25/1
  Input Demux/26 -> Multiply-Add 26/1
  Input Demux/27 -> Multiply-Add 27/1
  Input Demux/28 -> Multiply-Add 28/1
  Input Demux/29 -> Multiply-Add 29/1
  Input Demux/30 -> Multiply-Add 30/1
  Input Demux/31 -> Multiply-Add 31/1
  Input Demux/32 -> Multiply-Add 32/1
  Input Demux/33 -> Multiply-Add 33/1
  Input Demux/34 -> Multiply-Add 34/1
  Input Demux/35 -> Multiply-Add 35/1
  Input Demux/36 -> Multiply-Add 36/1
  Input Demux/37 -> Multiply-Add 37/1
  Input Demux/38 -> Multiply-Add 38/1
  Input Demux/39 -> Multiply-Add 39/1
  Input Demux/40 -> Multiply-Add 40/1
  Input Demux/41 -> Multiply-Add 41/1
  Input Demux/42 -> Multiply-Add 42/1
  Input Demux/43 -> Multiply-Add 43/1
  Input Demux/44 -> Multiply-Add 44/1
  Input Demux/45 -> Multiply-Add 45/1
  Input Demux/46 -> Multiply-Add 46/1
  Input Demux/47 -> Multiply-Add 47/1
  Input Demux/48 -> Multiply-Add 48/1
  Input Demux/49 -> Multiply-Add 49/1
  Input Demux/50 -> Multiply-Add 50/1
  Input Demux/51 -> Multiply-Add 51/1
  Input Demux/52 -> Multiply-Add 52/1
  Input Demux/53 -> Multiply-Add 53/1
  Input Demux/54 -> Multiply-Add 54/1
  Input Demux/55 -> Multiply-Add 55/1
  Input Demux/56 -> Multiply-Add 56/1
  Input Demux/57 -> Multiply-Add 57/1
  Input Demux/58 -> Multiply-Add 58/1
  Input Demux/59 -> Multiply-Add 59/1
  Input Demux/60 -> Multiply-Add 60/1
  c1/1 -> [c1]
  c2/1 -> [c2]
  c0/1 -> Multiply-Add 1/3

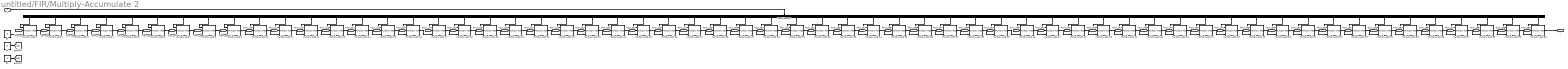
== system untitled/FIR/Multiply-Accumulate 2 ==
  x : Inport
  Input Demux : Demux  Outputs=60
  Multiply-Add {1..60} (60 alike) : filter_library/Multiply-Add  SystemSampleTime=-1
      settings: SourceProductName=Filter Library
  c0 : Constant  Value=0  OutDataTypeStr=fixdt(1, 12, 7)  SampleTime=1
  c1 : Constant  Value=-1  OutDataTypeStr=fixdt(1, 12, 7)  SampleTime=1
  c2 : Constant  OutDataTypeStr=fixdt(1, 12, 7)  SampleTime=1
  y : Outport
  wires:
  [c1] -> Multiply-Add 1/2
  [c1] -> Multiply-Add 2/2
  [c2] -> Multiply-Add 3/2
  [c2] -> Multiply-Add 4/2
  [c2] -> Multiply-Add 5/2
  [c1] -> Multiply-Add 6/2
  [c1] -> Multiply-Add 7/2
  [c2] -> Multiply-Add 8/2
  [c2] -> Multiply-Add 9/2
  [c1] -> Multiply-Add 10/2
  [c1] -> Multiply-Add 11/2
  [c1] -> Multiply-Add 12/2
  [c1] -> Multiply-Add 13/2
  [c1] -> Multiply-Add 14/2
  [c1] -> Multiply-Add 15/2
  [c1] -> Multiply-Add 16/2
  [c2] -> Multiply-Add 17/2
  [c2] -> Multiply-Add 18/2
  [c1] -> Multiply-Add 19/2
  [c1] -> Multiply-Add 20/2
  [c2] -> Multiply-Add 21/2
  [c1] -> Multiply-Add 22/2
  [c1] -> Multiply-Add 23/2
  [c1] -> Multiply-Add 24/2
  [c2] -> Multiply-Add 25/2
  [c1] -> Multiply-Add 26/2
  [c2] -> Multiply-Add 27/2
  [c1] -> Multiply-Add 28/2
  [c2] -> Multiply-Add 29/2
  [c1] -> Multiply-Add 30/2
  [c1] -> Multiply-Add 31/2
  [c2] -> Multiply-Add 32/2
  [c2] -> Multiply-Add 33/2
  [c2] -> Multiply-Add 34/2
  [c1] -> Multiply-Add 35/2
  [c1] -> Multiply-Add 36/2
  [c1] -> Multiply-Add 37/2
  [c2] -> Multiply-Add 38/2
  [c2] -> Multiply-Add 39/2
  [c2] -> Multiply-Add 40/2
  [c2] -> Multiply-Add 41/2
  [c1] -> Multiply-Add 42/2
  [c1] -> Multiply-Add 43/2
  [c2] -> Multiply-Add 44/2
  [c1] -> Multiply-Add 45/2
  [c1] -> Multiply-Add 46/2
  [c2] -> Multiply-Add 47/2
  [c1] -> Multiply-Add 48/2
  [c1] -> Multiply-Add 49/2
  [c1] -> Multiply-Add 50/2
  [c2] -> Multiply-Add 51/2
  [c1] -> Multiply-Add 52/2
  [c1] -> Multiply-Add 53/2
  [c2] -> Multiply-Add 54/2
  [c2] -> Multiply-Add 55/2
  [c1] -> Multiply-Add 56/2
  [c2] -> Multiply-Add 57/2
  [c2] -> Multiply-Add 58/2
  [c2] -> Multiply-Add 59/2
  [c2] -> Multiply-Add 60/2
  Multiply-Add 1/1 -> Multiply-Add 2/3
  Multiply-Add 2/1 -> Multiply-Add 3/3
  Multiply-Add 3/1 -> Multiply-Add 4/3
  Multiply-Add 4/1 -> Multiply-Add 5/3
  Multiply-Add 5/1 -> Multiply-Add 6/3
  Multiply-Add 6/1 -> Multiply-Add 7/3
  Multiply-Add 7/1 -> Multiply-Add 8/3
  Multiply-Add 8/1 -> Multiply-Add 9/3
  Multiply-Add 9/1 -> Multiply-Add 10/3
  Multiply-Add 10/1 -> Multiply-Add 11/3
  Multiply-Add 11/1 -> Multiply-Add 12/3
  Multiply-Add 12/1 -> Multiply-Add 13/3
  Multiply-Add 13/1 -> Multiply-Add 14/3
  Multiply-Add 14/1 -> Multiply-Add 15/3
  Multiply-Add 15/1 -> Multiply-Add 16/3
  Multiply-Add 16/1 -> Multiply-Add 17/3
  Multiply-Add 17/1 -> Multiply-Add 18/3
  Multiply-Add 18/1 -> Multiply-Add 19/3
  Multiply-Add 19/1 -> Multiply-Add 20/3
  Multiply-Add 20/1 -> Multiply-Add 21/3
  Multiply-Add 21/1 -> Multiply-Add 22/3
  Multiply-Add 22/1 -> Multiply-Add 23/3
  Multiply-Add 23/1 -> Multiply-Add 24/3
  Multiply-Add 24/1 -> Multiply-Add 25/3
  Multiply-Add 25/1 -> Multiply-Add 26/3
  Multiply-Add 26/1 -> Multiply-Add 27/3
  Multiply-Add 27/1 -> Multiply-Add 28/3
  Multiply-Add 28/1 -> Multiply-Add 29/3
  Multiply-Add 29/1 -> Multiply-Add 30/3
  Multiply-Add 30/1 -> Multiply-Add 31/3
  Multiply-Add 31/1 -> Multiply-Add 32/3
  Multiply-Add 32/1 -> Multiply-Add 33/3
  Multiply-Add 33/1 -> Multiply-Add 34/3
  Multiply-Add 34/1 -> Multiply-Add 35/3
  Multiply-Add 35/1 -> Multiply-Add 36/3
  Multiply-Add 36/1 -> Multiply-Add 37/3
  Multiply-Add 37/1 -> Multiply-Add 38/3
  Multiply-Add 38/1 -> Multiply-Add 39/3
  Multiply-Add 39/1 -> Multiply-Add 40/3
  Multiply-Add 40/1 -> Multiply-Add 41/3
  Multiply-Add 41/1 -> Multiply-Add 42/3
  Multiply-Add 42/1 -> Multiply-Add 43/3
  Multiply-Add 43/1 -> Multiply-Add 44/3
  Multiply-Add 44/1 -> Multiply-Add 45/3
  Multiply-Add 45/1 -> Multiply-Add 46/3
  Multiply-Add 46/1 -> Multiply-Add 47/3
  Multiply-Add 47/1 -> Multiply-Add 48/3
  Multiply-Add 48/1 -> Multiply-Add 49/3
  Multiply-Add 49/1 -> Multiply-Add 50/3
  Multiply-Add 50/1 -> Multiply-Add 51/3
  Multiply-Add 51/1 -> Multiply-Add 52/3
  Multiply-Add 52/1 -> Multiply-Add 53/3
  Multiply-Add 53/1 -> Multiply-Add 54/3
  Multiply-Add 54/1 -> Multiply-Add 55/3
  Multiply-Add 55/1 -> Multiply-Add 56/3
  Multiply-Add 56/1 -> Multiply-Add 57/3
  Multiply-Add 57/1 -> Multiply-Add 58/3
  Multiply-Add 58/1 -> Multiply-Add 59/3
  Multiply-Add 59/1 -> Multiply-Add 60/3
  Multiply-Add 60/1 -> y/1
  x/1 -> Input Demux/1
  Input Demux/1 -> Multiply-Add 1/1
  Input Demux/2 -> Multiply-Add 2/1
  Input Demux/3 -> Multiply-Add 3/1
  Input Demux/4 -> Multiply-Add 4/1
  Input Demux/5 -> Multiply-Add 5/1
  Input Demux/6 -> Multiply-Add 6/1
  Input Demux/7 -> Multiply-Add 7/1
  Input Demux/8 -> Multiply-Add 8/1
  Input Demux/9 -> Multiply-Add 9/1
  Input Demux/10 -> Multiply-Add 10/1
  Input Demux/11 -> Multiply-Add 11/1
  Input Demux/12 -> Multiply-Add 12/1
  Input Demux/13 -> Multiply-Add 13/1
  Input Demux/14 -> Multiply-Add 14/1
  Input Demux/15 -> Multiply-Add 15/1
  Input Demux/16 -> Multiply-Add 16/1
  Input Demux/17 -> Multiply-Add 17/1
  Input Demux/18 -> Multiply-Add 18/1
  Input Demux/19 -> Multiply-Add 19/1
  Input Demux/20 -> Multiply-Add 20/1
  Input Demux/21 -> Multiply-Add 21/1
  Input Demux/22 -> Multiply-Add 22/1
  Input Demux/23 -> Multiply-Add 23/1
  Input Demux/24 -> Multiply-Add 24/1
  Input Demux/25 -> Multiply-Add 25/1
  Input Demux/26 -> Multiply-Add 26/1
  Input Demux/27 -> Multiply-Add 27/1
  Input Demux/28 -> Multiply-Add 28/1
  Input Demux/29 -> Multiply-Add 29/1
  Input Demux/30 -> Multiply-Add 30/1
  Input Demux/31 -> Multiply-Add 31/1
  Input Demux/32 -> Multiply-Add 32/1
  Input Demux/33 -> Multiply-Add 33/1
  Input Demux/34 -> Multiply-Add 34/1
  Input Demux/35 -> Multiply-Add 35/1
  Input Demux/36 -> Multiply-Add 36/1
  Input Demux/37 -> Multiply-Add 37/1
  Input Demux/38 -> Multiply-Add 38/1
  Input Demux/39 -> Multiply-Add 39/1
  Input Demux/40 -> Multiply-Add 40/1
  Input Demux/41 -> Multiply-Add 41/1
  Input Demux/42 -> Multiply-Add 42/1
  Input Demux/43 -> Multiply-Add 43/1
  Input Demux/44 -> Multiply-Add 44/1
  Input Demux/45 -> Multiply-Add 45/1
  Input Demux/46 -> Multiply-Add 46/1
  Input Demux/47 -> Multiply-Add 47/1
  Input Demux/48 -> Multiply-Add 48/1
  Input Demux/49 -> Multiply-Add 49/1
  Input Demux/50 -> Multiply-Add 50/1
  Input Demux/51 -> Multiply-Add 51/1
  Input Demux/52 -> Multiply-Add 52/1
  Input Demux/53 -> Multiply-Add 53/1
  Input Demux/54 -> Multiply-Add 54/1
  Input Demux/55 -> Multiply-Add 55/1
  Input Demux/56 -> Multiply-Add 56/1
  Input Demux/57 -> Multiply-Add 57/1
  Input Demux/58 -> Multiply-Add 58/1
  Input Demux/59 -> Multiply-Add 59/1
  Input Demux/60 -> Multiply-Add 60/1
  c1/1 -> [c1]
  c2/1 -> [c2]
  c0/1 -> Multiply-Add 1/3
